simulink model "Farm_FaultBottomBar"  (R2019a)
(part 3 of 28)

  BusC3/LConn3 -- Three-Phase Breaker 10/RConn3 -- Three-Phase Breaker 22/LConn3
  Three-Phase Breaker 10/RConn1 -- Three-Phase Breaker 22/LConn1 -- BusC3/LConn1
  Three-Phase Breaker 11/RConn1 -- " 3"/LConn1
  Three-Phase Breaker 11/RConn2 -- " 3"/LConn2
  Three-Phase Breaker 11/RConn3 -- " 3"/LConn3
  Three-Phase Breaker 23/LConn3 -- BusC8/RConn3 -- Series RLC Load2/LConn1 -- Three-Phase Breaker 11/LConn3
  Three-Phase Breaker 12/LConn2 -- BusC4/RConn2
  Three-Phase Breaker 14/RConn2 -- " 4"/LConn2
  5 km series17/RConn1 -- Wind Type IV Detailed v2.1 - 14/LConn1
  Three-Phase Breaker 13/RConn3 -- BusC4/LConn3 -- Three-Phase Breaker 22/RConn3
  5 km series17/LConn3 -- Three-Phase Breaker 12/RConn3
  5 km series17/RConn2 -- Wind Type IV Detailed v2.1 - 14/LConn2
  Three-Phase Breaker 13/RConn2 -- BusC4/LConn2 -- Three-Phase Breaker 22/RConn2
  5 km series17/LConn2 -- Three-Phase Breaker 12/RConn2
  Three-Phase Breaker 13/RConn1 -- BusC4/LConn1 -- Three-Phase Breaker 22/RConn1
  Three-Phase Breaker 13/LConn2 -- " 4"/RConn2
  Three-Phase Breaker 14/RConn3 -- " 4"/LConn3
  Three-Phase Breaker 13/LConn3 -- " 4"/RConn3
  Three-Phase Breaker 14/RConn1 -- " 4"/LConn1
  5 km series17/RConn3 -- Wind Type IV Detailed v2.1 - 14/LConn3
  Three-Phase Breaker 13/LConn1 -- " 4"/RConn1
  5 km series17/LConn1 -- Three-Phase Breaker 12/RConn1
  Three-Phase Breaker 23/RConn1 -- Series RLC Load3/LConn1 -- Three-Phase Breaker 14/LConn1 -- BusC9/RConn1
  Three-Phase Breaker 23/RConn2 -- BusC9/RConn2 -- Series RLC Load4/LConn1 -- Three-Phase Breaker 14/LConn2
  Three-Phase Breaker 23/RConn3 -- Series RLC Load5/LConn1 -- Three-Phase Breaker 14/LConn3 -- BusC9/RConn3
  BusC6/RConn3 -- Three-Phase Breaker 27/LConn3
  Three-Phase Breaker 27/LConn1 -- BusC6/RConn1
  Three-Phase Breaker 27/LConn2 -- BusC6/RConn2
  Three-Phase Breaker 39/LConn3 -- Series RLC Load8/LConn1 -- Three-Phase Breaker 26/LConn3 -- BusC10/RConn3
  BusC5/RConn2 -- Three-Phase Breaker 41/LConn2
  BusC6/LConn3 -- Three-Phase Breaker 28/RConn3 -- Three-Phase Breaker 38/RConn3
  BusC5/LConn2 -- Three-Phase Breaker 25/RConn2 -- Three-Phase Breaker 38/LConn2
  Three-Phase Breaker 28/RConn1 -- BusC6/LConn1 -- Three-Phase Breaker 38/RConn1
  Three-Phase Breaker 41/LConn3 -- BusC5/RConn3
  Three-Phase Breaker 39/LConn2 -- BusC10/RConn2 -- Three-Phase Breaker 26/LConn2 -- Series RLC Load7/LConn1
  Three-Phase Breaker 28/RConn2 -- Three-Phase Breaker 38/RConn2 -- BusC6/LConn2
  BusC5/LConn3 -- Three-Phase Breaker 25/RConn3 -- Three-Phase Breaker 38/LConn3
  BusC5/LConn1 -- Three-Phase Breaker 25/RConn1 -- Three-Phase Breaker 38/LConn1
  Three-Phase Breaker 39/LConn1 -- Series RLC Load6/LConn1 -- Three-Phase Breaker 26/LConn1 -- BusC10/RConn1
  5 km series28/LConn2 -- Three-Phase Breaker 27/RConn2
  Three-Phase Breaker 26/RConn2 -- " 5"/LConn2
  Three-Phase Breaker 39/RConn2 -- Series RLC Load10/LConn1 -- Three-Phase Breaker 29/LConn2 -- BusC11/RConn2
  Three-Phase Breaker 29/RConn1 -- " 6"/LConn1
  5 km series28/RConn3 -- Wind Type IV Detailed v2.1 - 24/LConn3
  Three-Phase Breaker 28/LConn1 -- " 6"/RConn1
  Three-Phase Breaker 28/LConn3 -- " 6"/RConn3
  Three-Phase Breaker 28/LConn2 -- " 6"/RConn2
  Three-Phase Breaker 39/RConn1 -- Series RLC Load9/LConn1 -- Three-Phase Breaker 29/LConn1 -- BusC11/RConn1
  5 km series28/RConn1 -- Wind Type IV Detailed v2.1 - 24/LConn1
  5 km series28/RConn2 -- Wind Type IV Detailed v2.1 - 24/LConn2
  Three-Phase Breaker 39/RConn3 -- Series RLC Load11/LConn1 -- Three-Phase Breaker 29/LConn3 -- BusC11/RConn3
  Three-Phase Breaker 29/RConn2 -- " 6"/LConn2
  5 km series34/RConn2 -- Wind Type IV Detailed v2.1 - 33/LConn2
  5 km series34/RConn1 -- Wind Type IV Detailed v2.1 - 33/LConn1
  5 km series28/LConn1 -- Three-Phase Breaker 27/RConn1
  Three-Phase Breaker 25/LConn2 -- " 5"/RConn2
  Three-Phase Breaker 29/RConn3 -- " 6"/LConn3
  5 km series34/RConn3 -- Wind Type IV Detailed v2.1 - 33/LConn3
  5 km series34/LConn1 -- Three-Phase Breaker 41/RConn1
  5 km series28/LConn3 -- Three-Phase Breaker 27/RConn3
  Three-Phase Breaker 26/RConn3 -- " 5"/LConn3
  Three-Phase Breaker 26/RConn1 -- " 5"/LConn1
  Three-Phase Breaker 25/LConn3 -- " 5"/RConn3
  5 km series34/LConn3 -- Three-Phase Breaker 41/RConn3
  Three-Phase Breaker 25/LConn1 -- " 5"/RConn1
  5 km series34/LConn2 -- Three-Phase Breaker 41/RConn2
  Three-Phase Breaker 23/LConn2 -- BusC8/RConn2 -- Series RLC Load1/LConn1 -- Three-Phase Breaker 11/LConn2
  Three-Phase Breaker 23/LConn1 -- BusC8/RConn1 -- Three-Phase Breaker 11/LConn1 -- Series RLC Load/LConn1
  Three-Phase Breaker 8/RConn1 -- BusC11/LConn1
  Three-Phase Breaker 12/LConn1 -- BusC4/RConn1
  BusC4/RConn3 -- Three-Phase Breaker 12/LConn3
  Three-Phase Breaker 41/LConn1 -- BusC5/RConn1
  Three-Phase Breaker 6/RConn2 -- BusC10/LConn2
  Three-Phase Breaker 8/RConn3 -- BusC11/LConn3
  BusC10/LConn3 -- Three-Phase Breaker 6/RConn3
  Three-Phase Breaker 8/RConn2 -- BusC11/LConn2
  BusC10/LConn1 -- Three-Phase Breaker 6/RConn1
  5 km series3/RConn1 -- Three-Phase Breaker 1/LConn1
  5 km series3/RConn2 -- Three-Phase Breaker 1/LConn2
  5 km series3/RConn3 -- Three-Phase Breaker 1/LConn3
  Three-Phase Breaker 2/RConn1 -- 5 km series3/LConn1
  Three-Phase Breaker 2/RConn2 -- 5 km series3/LConn2
  Three-Phase Breaker 2/RConn3 -- 5 km series3/LConn3
  Three-Phase Breaker 1/RConn1 -- BusC8/LConn1
  Three-Phase Breaker 1/RConn2 -- BusC8/LConn2
  Three-Phase Breaker 1/RConn3 -- BusC8/LConn3
  BusC12/RConn1 -- Three-Phase Breaker 2/LConn1
  BusC12/RConn2 -- Three-Phase Breaker 2/LConn2
  BusC12/RConn3 -- Three-Phase Breaker 2/LConn3
  Three-Phase Breaker 5/RConn3 -- 5 km series4/LConn3
  Three-Phase Breaker 5/RConn1 -- 5 km series4/LConn1
  5 km series4/RConn2 -- Three-Phase Breaker 3/LConn2
  5 km series4/RConn1 -- Three-Phase Breaker 3/LConn1
  BusC13/RConn1 -- Three-Phase Breaker 5/LConn1
  5 km series4/RConn3 -- Three-Phase Breaker 3/LConn3
  BusC13/RConn3 -- Three-Phase Breaker 5/LConn3
  BusC13/RConn2 -- Three-Phase Breaker 5/LConn2
  Three-Phase Breaker 5/RConn2 -- 5 km series4/LConn2
  Three-Phase Breaker 7/RConn3 -- 5 km series5/LConn3
  Three-Phase Breaker 7/RConn1 -- 5 km series5/LConn1
  5 km series5/RConn2 -- Three-Phase Breaker 6/LConn2
  5 km series5/RConn1 -- Three-Phase Breaker 6/LConn1
  BusC14/RConn1 -- Three-Phase Breaker 7/LConn1
  5 km series5/RConn3 -- Three-Phase Breaker 6/LConn3
  BusC14/RConn3 -- Three-Phase Breaker 7/LConn3
  BusC14/RConn2 -- Three-Phase Breaker 7/LConn2
  Three-Phase Breaker 7/RConn2 -- 5 km series5/LConn2
  Three-Phase Breaker 15/RConn3 -- 5 km series6/LConn3
  Three-Phase Breaker 15/RConn1 -- 5 km series6/LConn1
  5 km series6/RConn2 -- Three-Phase Breaker 8/LConn2
  5 km series6/RConn1 -- Three-Phase Breaker 8/LConn1
  BusC15/RConn1 -- Three-Phase Breaker 15/LConn1
  5 km series6/RConn3 -- Three-Phase Breaker 8/LConn3
  BusC15/RConn3 -- Three-Phase Breaker 15/LConn3
  BusC15/RConn2 -- Three-Phase Breaker 15/LConn2
  Three-Phase Breaker 15/RConn2 -- 5 km series6/LConn2
  BusC12/LConn1 -- BusC15/LConn1 -- BusC14/LConn1 -- BusC13/LConn1 -- BusC7/RConn1
  BusC12/LConn2 -- BusC15/LConn2 -- BusC14/LConn2 -- BusC13/LConn2 -- BusC7/RConn2
  BusC12/LConn3 -- BusC14/LConn3 -- BusC15/LConn3 -- BusC13/LConn3 -- BusC7/RConn3
  5 km series7/RConn2 -- Three-Phase Breaker 16/LConn2
  5 km series7/RConn1 -- Three-Phase Breaker 16/LConn1
  Three-Phase Breaker 17/RConn3 -- 5 km series7/LConn3
  BusC16/RConn3 -- Three-Phase Breaker 17/LConn3
  BusC16/RConn1 -- Three-Phase Breaker 17/LConn1
  Three-Phase Breaker 17/RConn1 -- 5 km series7/LConn1
  5 km series7/RConn3 -- Three-Phase Breaker 16/LConn3
  BusC16/RConn2 -- Three-Phase Breaker 17/LConn2
  Three-Phase Breaker 17/RConn2 -- 5 km series7/LConn2
  5 km series8/RConn2 -- Three-Phase Breaker 18/LConn2
  5 km series8/RConn1 -- Three-Phase Breaker 18/LConn1
  Three-Phase Breaker 19/RConn3 -- 5 km series8/LConn3
  BusC17/RConn3 -- Three-Phase Breaker 19/LConn3
  BusC17/RConn1 -- Three-Phase Breaker 19/LConn1
  Three-Phase Breaker 19/RConn1 -- 5 km series8/LConn1
  5 km series8/RConn3 -- Three-Phase Breaker 18/LConn3
  BusC17/RConn2 -- Three-Phase Breaker 19/LConn2
  Three-Phase Breaker 19/RConn2 -- 5 km series8/LConn2
  Three-Phase Breaker 16/RConn1 -- Three-Phase Breaker 18/RConn1 -- BusC7/LConn1
  Three-Phase Breaker 16/RConn2 -- Three-Phase Breaker 18/RConn2 -- BusC7/LConn2
  Three-Phase Breaker 16/RConn3 -- Three-Phase Breaker 18/RConn3 -- BusC7/LConn3
  BusC17/LConn1 -- BusC16/LConn1 -- BusC18/RConn1
  BusC16/LConn2 -- BusC18/RConn2 -- BusC17/LConn2
  BusC17/LConn3 -- BusC18/RConn3 -- BusC16/LConn3
  BusC9/LConn1 -- Three-Phase Breaker 3/RConn1
  BusC9/LConn2 -- Three-Phase Breaker 3/RConn2
  BusC9/LConn3 -- Three-Phase Breaker 3/RConn3
  BusC18/LConn2 -- 2500 MVA X0/X1=2/RConn2
  2500 MVA X0/X1=2/RConn1 -- BusC18/LConn1
  2500 MVA X0/X1=2/RConn3 -- BusC18/LConn3
  Ground3/LConn1 -- Series RLC Load/RConn1
  Ground4/LConn1 -- Series RLC Load1/RConn1
  Ground5/LConn1 -- Series RLC Load2/RConn1
  Ground7/LConn1 -- Series RLC Load4/RConn1
  Ground6/LConn1 -- Series RLC Load3/RConn1
  Ground8/LConn1 -- Series RLC Load5/RConn1
  Ground10/LConn1 -- Series RLC Load7/RConn1
  Ground9/LConn1 -- Series RLC Load6/RConn1
  Ground11/LConn1 -- Series RLC Load8/RConn1
  Ground13/LConn1 -- Series RLC Load10/RConn1
  Ground12/LConn1 -- Series RLC Load9/RConn1
  Ground14/LConn1 -- Series RLC Load11/RConn1
  Three-Phase Fault1/LConn1 -- 5 km series11/LConn1 -- BusC3/RConn1
